simulink model "Sistema"  (R2023a)
settings: Solver=VariableStepAuto  StartTime=0.0  StopTime=2  RelTol=1e-3
libraries: visiontextngfix x4
settings Model: Creator=a2150336  LastModifiedBy=a2150336

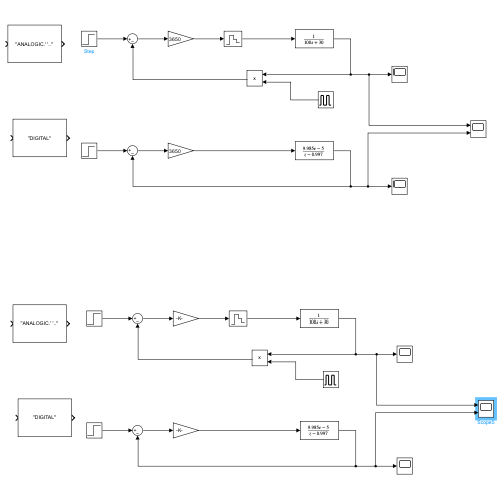
[thumbnail: Simulink's stored preview of the top-level diagram]
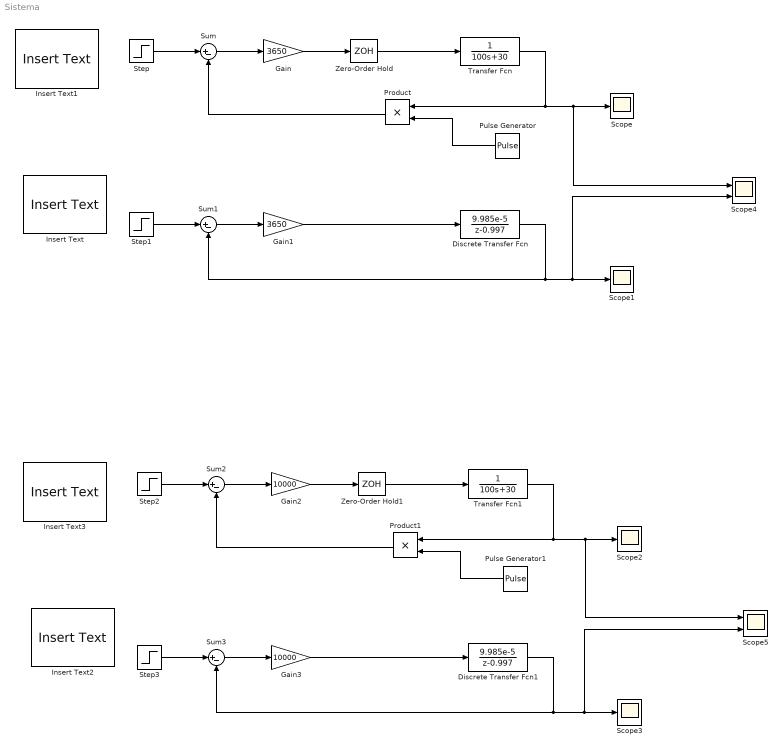
== system Sistema ==
  Discrete Transfer Fcn : DiscreteTransferFcn  Numerator=[9.985e-5]  Denominator=[1 -0.997]  SampleTime=0.01
  Discrete Transfer Fcn1 : DiscreteTransferFcn  Numerator=[9.985e-5]  Denominator=[1 -0.997]  SampleTime=0.01
  Gain : Gain  Gain=3650
  Gain1 : Gain  Gain=3650
  Gain2 : Gain  Gain=10000
  Gain3 : Gain  Gain=10000
  Insert Text : visiontextngfix/Insert Text  inputType=Obsolete  theText='DIGITAL'  getTextLocFrom=Specify via dialog  textLoc=[1 1]  getTextColorFrom=Specify via dialog  textColor=[0 0 0]  getTextIntensityFrom=Specify via dialog  textIntensity=0  getTextOpacityFrom=Specify via dialog  textOpacity=1.0  dummyVar2=0  dummyVar3=0  dummyVar4=0  imagePorts=One multidimensional signal  isInputTransposed=off  fontFace=LucidaSansRegular  dummyVar1=0  blockFontSize=12  antiAliased=on
  Insert Text1 : visiontextngfix/Insert Text  inputType=Obsolete  theText='ANALOGICO COM CONVERSOR A/D D/A'  getTextLocFrom=Specify via dialog  textLoc=[1 1]  getTextColorFrom=Specify via dialog  textColor=[0 0 0]  getTextIntensityFrom=Specify via dialog  textIntensity=0  getTextOpacityFrom=Specify via dialog  textOpacity=1.0  dummyVar2=0  dummyVar3=0  dummyVar4=0  imagePorts=One multidimensional signal  isInputTransposed=off  fontFace=LucidaSansRegular  dummyVar1=0  blockFontSize=12  antiAliased=on
  Insert Text2 : visiontextngfix/Insert Text  inputType=Obsolete  theText='DIGITAL'  getTextLocFrom=Specify via dialog  textLoc=[1 1]  getTextColorFrom=Specify via dialog  textColor=[0 0 0]  getTextIntensityFrom=Specify via dialog  textIntensity=0  getTextOpacityFrom=Specify via dialog  textOpacity=1.0  dummyVar2=0  dummyVar3=0  dummyVar4=0  imagePorts=One multidimensional signal  isInputTransposed=off  fontFace=LucidaSansRegular  dummyVar1=0  blockFontSize=12  antiAliased=on
  Insert Text3 : visiontextngfix/Insert Text  inputType=Obsolete  theText='ANALOGICO COM CONVERSOR A/D D/A'  getTextLocFrom=Specify via dialog  textLoc=[1 1]  getTextColorFrom=Specify via dialog  textColor=[0 0 0]  getTextIntensityFrom=Specify via dialog  textIntensity=0  getTextOpacityFrom=Specify via dialog  textOpacity=1.0  dummyVar2=0  dummyVar3=0  dummyVar4=0  imagePorts=One multidimensional signal  isInputTransposed=off  fontFace=LucidaSansRegular  dummyVar1=0  blockFontSize=12  antiAliased=on
  Product : Product
  Product1 : Product
  Pulse Generator : DiscretePulseGenerator  PulseType=Time based  Period=0.01  PulseWidth=0.1
  Pulse Generator1 : DiscretePulseGenerator  PulseType=Time based  Period=0.01  PulseWidth=0.1
  Scope{,1..3} (4 alike) : Scope
  Scope4 : Scope  NumInputPorts=2
  Scope5 : Scope  NumInputPorts=2
  Step{,1..3} (4 alike) : Step  SampleTime=0
  Sum{,1..3} (4 alike) : Sum  Inputs=|+-
  Transfer Fcn : TransferFcn  Denominator=[100 30]
  Transfer Fcn1 : TransferFcn  Denominator=[100 30]
  Zero-Order Hold : ZeroOrderHold  SampleTime=0.01
  Zero-Order Hold1 : ZeroOrderHold  SampleTime=0.01
  wires:
  Sum/1 -> Gain/1
  Gain/1 -> Zero-Order Hold/1
  Zero-Order Hold/1 -> Transfer Fcn/1
  Transfer Fcn/1 -> Product/1, Scope4/1, Scope/1
  Product/1 -> Sum/2
  Pulse Generator/1 -> Product/2
  Step/1 -> Sum/1
  Gain1/1 -> Discrete Transfer Fcn/1
  Step1/1 -> Sum1/1
  Discrete Transfer Fcn/1 -> Sum1/2, Scope4/2, Scope1/1
  Sum1/1 -> Gain1/1
  Step3/1 -> Sum3/1
  Sum3/1 -> Gain3/1
  Pulse Generator1/1 -> Product1/2
  Zero-Order Hold1/1 -> Transfer Fcn1/1
  Step2/1 -> Sum2/1
  Sum2/1 -> Gain2/1
  Gain3/1 -> Discrete Transfer Fcn1/1
  Gain2/1 -> Zero-Order Hold1/1
  Product1/1 -> Sum2/2
  Discrete Transfer Fcn1/1 -> Sum3/2, Scope5/2, Scope3/1
  Transfer Fcn1/1 -> Product1/1, Scope5/1, Scope2/1
